simulink model "Clarke_Park_Transformations"  (R2022a)
settings: Solver=ode1  StartTime=0.0  StopTime=10  FixedStep=0.001  RelTol=1e-3
libraries: mcbcontrolslib x2
settings Model: Creator=LabPC  LastModifiedBy=LabPC

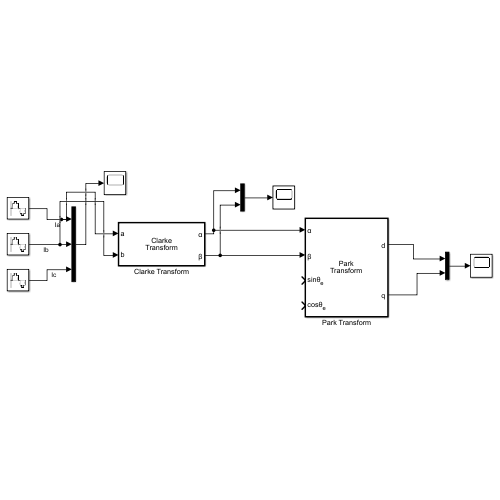
[thumbnail: Simulink's stored preview of the top-level diagram]
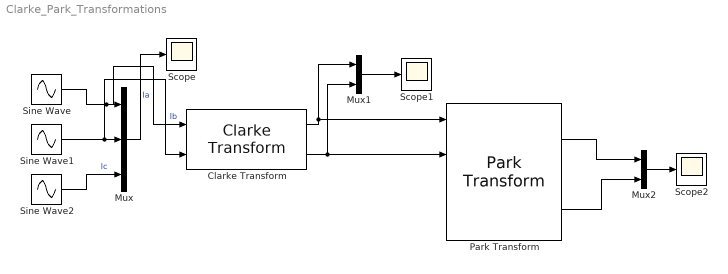
== system Clarke_Park_Transformations ==
  Clarke Transform : mcbcontrolslib/Clarke Transform  VariantControl=Variant2
  Mux : Mux  Inputs=3
  Mux1 : Mux  Inputs=2
  Mux2 : Mux  Inputs=2
  Park Transform : mcbcontrolslib/Park Transform  AxisAlignment=D-axis
      settings: SourceProductBaseCode=MT
  Scope : Scope
  Scope1 : Scope
  Scope2 : Scope
  Sine Wave : Sin  Amplitude=12  Frequency=2*pi*1  SampleTime=0.001  VectorParams1D=off
  Sine Wave1 : Sin  Amplitude=12  Frequency=2*pi*1  Phase=2*pi/3  SampleTime=0.001  VectorParams1D=off
  Sine Wave2 : Sin  Amplitude=12  Frequency=2*pi*1  Phase=-2*pi/3  SampleTime=0.001  VectorParams1D=off
  wires:
  Sine Wave/1 -> Clarke Transform/1, Mux/1  "Ia"
  Sine Wave1/1 -> Clarke Transform/2, Mux/2  "Ib"
  Sine Wave2/1 -> Mux/3  "Ic"
  Mux/1 -> Scope/1
  Clarke Transform/2 -> Mux1/2, Park Transform/2
  Mux1/1 -> Scope1/1
  Mux2/1 -> Scope2/1
  Clarke Transform/1 -> Mux1/1, Park Transform/1
  Park Transform/1 -> Mux2/1
  Park Transform/2 -> Mux2/2
